simulink model "Loop_model"  (R2023b)
settings: Solver=ode5  StartTime=0.0  StopTime=1e4  RelTol=1e-3
values from neighbouring files (symbols this model uses):
  a = 6851.22197053    [IGRF13_2020.mat]    (also in complete_model.m; complete_model_main.m; loop_model.m; orbit_plot_report.m)
  alpha1 = 0.4    [IGRF13_2020.mat]    (also in complete_model.m = 0.05; complete_model_main.m; loop_model.m)
  alpha2 = 0.1    [IGRF13_2020.mat]    (also in complete_model.m = 0.15; complete_model_main.m; loop_model.m)
  alpha3 = 0.5    [IGRF13_2020.mat]    (also in complete_model.m = 0.8; complete_model_main.m; loop_model.m)
  bias_earth = [0.0282799758328 0.672423061801 0.739626573972]    [IGRF13_2020.mat]    (also in bias_good.mat = [0.12529783722 0.977879152241 0.167489747749]; complete_model.m = bias_earth./norm(bias_earth); loop_model.m = bias_earth./norm(bias_earth))
  bias_mag = [0.139359936806 0.414251479478 0.899430108326]    [IGRF13_2020.mat]    (also in bias_good.mat = [0.633137130131 0.601746707773 0.486865766031]; complete_model.m = bias_mag./norm(bias_mag); loop_model.m = bias_mag./norm(bias_mag))
  bias_sun = [0.56325131841 0.682189313334 0.466224938288]    [IGRF13_2020.mat]    (also in bias_good.mat = [0.711264013876 0.679091205187 0.181490048217]; complete_model.m = bias_sun./norm(bias_sun); loop_model.m = bias_sun./norm(bias_sun))
  e = 0.00183012221618    [IGRF13_2020.mat]    (also in complete_model.m; complete_model_main.m; loop_model.m; orbit_plot_report.m)
  FOV_earth = 0.575958653158    [IGRF13_2020.mat]    (also in complete_model.m = deg2rad(33); complete_model_main.m = deg2rad(33); loop_model.m = deg2rad(33))
  freq_acds = 30    [IGRF13_2020.mat]    (also in complete_model.m; loop_model.m)
  freq_act = 30    [IGRF13_2020.mat]    (also in complete_model.m; complete_model_main.m = 5; loop_model.m)
  freq_earth = 30    [IGRF13_2020.mat]    (also in complete_model.m; complete_model_main.m = 5; loop_model.m)
  freq_mag = 30    [IGRF13_2020.mat]    (also in complete_model.m; complete_model_main.m = 5; loop_model.m)
  freq_sun = 30    [IGRF13_2020.mat]    (also in complete_model.m; complete_model_main.m = 5; loop_model.m)
  gh = [-29404.8 -1450.9 4652.5 -2499.6 2982 -2991.6 1677 -734.6 1363.2 -2381.2 -82.1 1236.2 ... (195 elements, 195x1)]    [IGRF13_2020.mat]
  H0 = 2.98059244128e-05    [IGRF13_2020.mat]    (also in complete_model.m = sqrt(g01^2+g11^2+h11^2)*1e-9; complete_model_main.m = sqrt(g01^2+g11^2+h11^2)*1e-9; loop_model.m = sqrt(g01^2+g11^2+h11^2)*1e-9)
  I_ext = [22.9724026819  0  0; 0  7.77699984285  0; 0  0  23.1895034219]    [IGRF13_2020.mat]    (also in complete_model.m = diag([I1_ext I2_ext I3_ext]); loop_model.m = diag([I1_ext I2_ext I3_ext]))
  I_retr = [8.16666666667  0  0; 0  8.16666666667  0; 0  0  8.16666666667]    [IGRF13_2020.mat]    (also in complete_model.m = diag([I1_retr I2_retr I3_retr]); loop_model.m = diag([I1_retr I2_retr I3_retr]))
  I_wheel = 0.00636619772368    [IGRF13_2020.mat]    (also in complete_model.m; loop_model.m)
  Iinv_ext = [0.0435304923845  0  0; 0  0.128584289598  0; 0  0  0.0431229587718]    [IGRF13_2020.mat]    (also in complete_model.m = I_ext\eye(3); loop_model.m = I_ext\eye(3))
  Iinv_retr = [0.122448979592  0  0; 0  0.122448979592  0; 0  0  0.122448979592]    [IGRF13_2020.mat]    (also in complete_model.m = I_retr\eye(3); loop_model.m = I_retr\eye(3))
  incl = 0.200712863979    [IGRF13_2020.mat]    (also in complete_model.m = deg2rad(11.5); complete_model_main.m = deg2rad(11.5); loop_model.m = deg2rad(11.5))
  jb = [0.01 0.05 0.01]    [IGRF13_2020.mat]    (also in complete_model.m = [0.01; 0.05; 0.01]; complete_model_main.m = [0.01; 0.05; 0.01]; loop_model.m = [0.01; 0.05; 0.01])
  k_gain = 0.0363323388759    [IGRF13_2020.mat]    (also in complete_model.m = (4*pi/T) * (1 + sin(chsi)) * I1_retr; complete_model_main.m = (4*pi/T) * (1 + sin(chsi)) * min([I1, I2, I3]); loop_model.m = (4*pi/T) * (1 + sin(chsi)) * I1_retr)
  max_dip = 15    [IGRF13_2020.mat]    (also in complete_model.m; complete_model_main.m = 150; loop_model.m)
  max_hdot = 0.1    [IGRF13_2020.mat]    (also in complete_model.m; loop_model.m)
  mu = 398600.433    [IGRF13_2020.mat]    (also in complete_model.m = astroConstants(13); complete_model_main.m = astroConstants(13); loop_model.m = astroConstants(13); orbit_plot_report.m = astroConstants(13))
  n = 0.00111331183439    [IGRF13_2020.mat]    (also in complete_model.m = sqrt(mu/a^3); complete_model_main.m = sqrt(mu/a^3); loop_model.m = sqrt(mu/a^3); orbit_plot_report.m = sqrt(mu/a^3))
  noise_sd_mag = 1.18e-09    [IGRF13_2020.mat]    (also in complete_model.m; loop_model.m)
  omega0 = [0.06 0.06 0.06]    [IGRF13_2020.mat]    (also in complete_model.m = -0.06 + 0.12 * rand(3,1); complete_model_main.m = [0.01; 0.01; 0.01]*6; init_cond.mat = [-0.0472016675783 0.0554277697026 -0.0594438931039]; loop_model.m = 0.06 * ones(3,1))
  omegaE = 7.27220521664e-05    [IGRF13_2020.mat]    (also in complete_model.m = deg2rad(15)/3600; complete_model_main.m = deg2rad(15)/3600; loop_model.m = deg2rad(15)/3600)
  rs = [-16878165.0145 -134206589.72 -58177126.6728]    [IGRF13_2020.mat]    (also in complete_model.m = -rr; complete_model_main.m = -rr; loop_model.m = -rr; orbit_plot_report.m = -rr)
  Rt = 6371.01    [IGRF13_2020.mat]    (also in Terra_3D.m = 6378.1363; complete_model.m = astroConstants(23); complete_model_main.m = astroConstants(23); loop_model.m = astroConstants(23))
  s0 = [6.01405730572 3.04970514452 5.02831048374]    [IGRF13_2020.mat]    (also in buonnatale.mat = [2.59731710564 0.831637671153 -2.52872821404]; complete_model.m = 2*pi*rand(3,1); complete_model_main.m = -pi + 2 * pi * rand(3,1); init_cond.mat = [4.86890604626 5.13526758752 5.45816980916])
  tol = 0.2    [IGRF13_2020.mat]    (also in complete_model.m; complete_model_main.m; loop_model.m)
  w_sat = 628.318530718    [IGRF13_2020.mat]    (also in complete_model.m; loop_model.m)
undefined symbols (not defined in the file or in its folder): DiscIntNeverNeededParam, flag_h, magnitude, s_h, s_m, s_s, v_h, v_m, v_s
libraries: simulink x16, vrlib x9, matrix_library x7, cstextras x3, simulink_extras x1
(part 3 of 3)

== system Loop_model/Control/Slew Maneuver/Control Logic/Subsystem1 ==
  B_m : Inport
  u : Inport  Port=2
  Enable : EnablePort
  Assembly Matrix : Subsystem
  Constant : Constant  Value=0
  Constant1 : Constant  Value=0
  MATLAB Function : MATLAB Function  TreatAsAtomicUnit=on
  Selector : Selector  InputPortWidth=3  IndexOptions=Index vector (dialog)  Indices=2  OutputSizes=1
  Selector1 : Selector  InputPortWidth=3  IndexOptions=Index vector (dialog)  Indices=3  OutputSizes=1
  Selector2 : Selector  InputPortWidth=3  IndexOptions=Index vector (dialog)  Indices=1  OutputSizes=1
  Vector Concatenate : Concatenate  NumInputs=5
  Out1 : Outport
  wires:
  Assembly Matrix/1("Matrix ") -> MATLAB Function/1(A)
  B_m/1 -> Assembly Matrix/1(B_m)
  Selector1/1 -> Vector Concatenate/3
  Selector/1 -> Vector Concatenate/2
  Constant/1 -> Vector Concatenate/1
  Selector2/1 -> Vector Concatenate/4
  Constant1/1 -> Vector Concatenate/5
  MATLAB Function/1(x) -> Selector/1, Selector2/1, Selector1/1
  Vector Concatenate/1 -> Out1/1
  u/1 -> MATLAB Function/2(b)

== system Loop_model/Control/Slew Maneuver/compute alphadots/Discrete Derivative ==
  note: ( U(k) - U(k-1) )
  note: U(k)
  U : Inport
  Data Type Duplicate : DataTypeDuplicate  DisableCoverage=on  NumInputPorts=3
  Diff : Sum  Description=Add in CPU  Inputs=+-  OutMin=OutMin  OutMax=OutMax  OutDataTypeStr=diffDT
  TSamp : SampleTimeMath  DisableCoverage=on  TsampMathOp=/  weightValue=inverseGainval  TsampMathImp=Offline Scaling Adjustment
  UD : UnitDelay  Description=Store in Global RAM  DisableCoverage=on  InitialCondition=ICPrevScaledInput  SampleTime=-1  HasFrameUpgradeWarning=on
  Y : Outport  OutMin=OutMin  OutMax=OutMax  InitialOutput=0
  wires:
  U/1 -> TSamp/1
  UD/1 -> Diff/2, Data Type Duplicate/3  "U(k-1)"
  Diff/1 -> Y/1, Data Type Duplicate/1
  TSamp/1 -> UD/1, Diff/1, Data Type Duplicate/2

== system Loop_model/Control/Slew Maneuver/compute alphadots/Discrete Varying Lowpass ==
  u : Inport
  frequency : Inport  Port=2
  FOS : cstextras/DiscreteFirstOrderSection  VariantControl=(default)  Ts=Ts  w0=w0
  y : Outport  VectorParamsAs1DForOutWhenUnconnected=off
  wires:
  u/1 -> FOS/1
  frequency/1 -> FOS/2
  FOS/1 -> y/1

== system Loop_model/Control/Slew Maneuver/compute alphadots/Invert ==
  Matrix : Inport  PortDimensions=[3 3]
  Assertion : Assertion  AssertionFailFcn="disp('Matrix is singular.  No matrix inverse.')"
  Determinant of 3x3 Matrix : Subsystem
      settings: LibrarySourceBlock=|
      | sharedutil/Determinant of
      | 3x3 Matrix
  Product : Product  Inputs=/  Multiplication=Matrix(*)  SaturateOnIntegerOverflow=on  OutDataTypeStr=Inherit: Same as first input
  Matrix' : Outport  PortDimensions=[3 3]  VectorParamsAs1DForOutWhenUnconnected=off
  wires:
  Determinant of 3x3 Matrix/1(det) -> Assertion/1
  Product/1 -> Matrix'/1
  Matrix/1 -> Product/1, Determinant of 3x3 Matrix/1(Matrix)

== system Loop_model/Environment/Magnetic Field/compute Bn/compute m ==
  Clock : Clock
  Constant : Constant  Value=incl
  Constant1 : Constant  Value=omegaE
  Cos : Trigonometry  Operator=cos
  Cos1 : Trigonometry  Operator=cos
  Product : Product
  Product1 : Product
  Product2 : Product
  Scope : Scope
  Sin : Trigonometry
  Sin1 : Trigonometry
  Vector Concatenate : Concatenate  NumInputs=3
  m : Outport
  wires:
  Sin1/1 -> Product2/1
  Clock/1 -> Product/1
  Cos1/1 -> Product1/1
  Constant1/1 -> Product/2
  Product2/1 -> Vector Concatenate/2
  Sin/1 -> Product2/2, Product1/2
  Product/1 -> Sin1/1, Cos1/1
  Product1/1 -> Vector Concatenate/1
  Constant/1 -> Cos/1, Sin/1
  Vector Concatenate/1 -> m/1, Scope/1
  Cos/1 -> Vector Concatenate/3

== system Loop_model/Environment/Magnetic Field/compute Bn/norm ==
  rN : Inport
  Dot Product : DotProduct  OutDataTypeStr=Inherit: Inherit via internal rule
  Sqrt : Sqrt
  Out1 : Outport
  wires:
  rN/1 -> Dot Product/1, Dot Product/2
  Dot Product/1 -> Sqrt/1
  Sqrt/1 -> Out1/1

== system Loop_model/Kinematics/Kinematics 312/Euler angles/Subsystem ==
  In1 : Inport
  In2 : Inport  Port=2
  In3 : Inport  Port=3
  Cos : Trigonometry  Operator=cos
  Product : Product
  Product1 : Product
  Sin : Trigonometry
  Sum : Sum
  Out1 : Outport
  wires:
  In3/1 -> Sin/1, Cos/1
  In1/1 -> Product/1
  Cos/1 -> Product/2
  Sin/1 -> Product1/1
  In2/1 -> Product1/2
  Product/1 -> Sum/1
  Product1/1 -> Sum/2
  Sum/1 -> Out1/1

== system Loop_model/Kinematics/Kinematics 312/Euler angles/Subsystem1 ==
  In1 : Inport
  In2 : Inport  Port=2
  In3 : Inport  Port=3
  Cos : Trigonometry  Operator=cos
  Product : Product
  Product1 : Product
  Sin : Trigonometry
  Sum : Sum
  Out1 : Outport
  wires:
  Sum/1 -> Out1/1
  Product1/1 -> Sum/2
  Product/1 -> Sum/1
  In2/1 -> Product1/2
  Sin/1 -> Product1/1
  Cos/1 -> Product/2
  In1/1 -> Product/1
  In3/1 -> Cos/1, Sin/1

== system Loop_model/Kinematics/Kinematics 312/Euler angles/Subsystem2 ==
  In1 : Inport
  In2 : Inport  Port=2
  In3 : Inport  Port=3
  Cos : Trigonometry  Operator=cos
  Product : Product
  Product1 : Product
  Sin : Trigonometry
  Sum : Sum
  Out1 : Outport
  wires:
  In3/1 -> Sin/1, Cos/1
  In1/1 -> Product/1
  Cos/1 -> Product/2
  Sin/1 -> Product1/1
  In2/1 -> Product1/2
  Product/1 -> Sum/1
  Product1/1 -> Sum/2
  Sum/1 -> Out1/1

== system Loop_model/Kinematics/Kinematics 312/s_312 - A/R1 ==
  x : Inport
  Constant : Constant  Value=[1; 0; 0]
  Constant1 : Constant  Value=0
  Cos : Trigonometry  Operator=cos
  Gain : Gain  Gain=-1
  Matrix Concatenate : Concatenate  NumInputs=3  Mode=Multidimensional array  ConcatenateDimension=2
  Sin : Trigonometry
  Vector Concatenate : Concatenate  NumInputs=3
  Vector Concatenate1 : Concatenate  NumInputs=3
  R1 : Outport
  wires:
  Matrix Concatenate/1 -> R1/1
  x/1 -> Cos/1, Sin/1
  Vector Concatenate1/1 -> Matrix Concatenate/2
  Constant/1 -> Matrix Concatenate/1
  Vector Concatenate/1 -> Matrix Concatenate/3
  Constant1/1 -> Vector Concatenate/1, Vector Concatenate1/1
  Cos/1 -> Vector Concatenate/3, Vector Concatenate1/2
  Gain/1 -> Vector Concatenate1/3
  Sin/1 -> Vector Concatenate/2, Gain/1

== system Loop_model/Kinematics/Kinematics 312/s_312 - A/R2 ==
  x : Inport
  Constant : Constant  Value=[0; 1; 0]
  Constant1 : Constant  Value=0
  Cos : Trigonometry  Operator=cos
  Gain : Gain  Gain=-1
  Matrix Concatenate : Concatenate  NumInputs=3  Mode=Multidimensional array  ConcatenateDimension=2
  Sin : Trigonometry
  Vector Concatenate : Concatenate  NumInputs=3
  Vector Concatenate1 : Concatenate  NumInputs=3
  R2 : Outport
  wires:
  Vector Concatenate/1 -> Matrix Concatenate/1
  x/1 -> Sin/1, Cos/1
  Matrix Concatenate/1 -> R2/1
  Constant/1 -> Matrix Concatenate/2
  Vector Concatenate1/1 -> Matrix Concatenate/3
  Constant1/1 -> Vector Concatenate/2, Vector Concatenate1/2
  Cos/1 -> Vector Concatenate1/3, Vector Concatenate/1
  Sin/1 -> Gain/1, Vector Concatenate/3
  Gain/1 -> Vector Concatenate1/1

== system Loop_model/Kinematics/Kinematics 312/s_312 - A/R3 ==
  x : Inport
  Constant : Constant  Value=[0; 0; 1]
  Constant1 : Constant  Value=0
  Cos : Trigonometry  Operator=cos
  Gain : Gain  Gain=-1
  Matrix Concatenate : Concatenate  NumInputs=3  Mode=Multidimensional array  ConcatenateDimension=2
  Sin : Trigonometry
  Vector Concatenate : Concatenate  NumInputs=3
  Vector Concatenate1 : Concatenate  NumInputs=3
  R3 : Outport
  wires:
  Vector Concatenate/1 -> Matrix Concatenate/1
  Sin/1 -> Vector Concatenate1/1, Gain/1
  Cos/1 -> Vector Concatenate1/2, Vector Concatenate/1
  Constant/1 -> Matrix Concatenate/3
  Gain/1 -> Vector Concatenate/2
  Vector Concatenate1/1 -> Matrix Concatenate/2
  x/1 -> Sin/1, Cos/1
  Constant1/1 -> Vector Concatenate/3, Vector Concatenate1/3
  Matrix Concatenate/1 -> R3/1

== system Loop_model/Kinematics/Kinematics 312/s_313 - A/R1 ==
  x : Inport
  Constant : Constant  Value=[1; 0; 0]
  Constant1 : Constant  Value=0
  Cos : Trigonometry  Operator=cos
  Gain : Gain  Gain=-1
  Matrix Concatenate : Concatenate  NumInputs=3  Mode=Multidimensional array  ConcatenateDimension=2
  Sin : Trigonometry
  Vector Concatenate : Concatenate  NumInputs=3
  Vector Concatenate1 : Concatenate  NumInputs=3
  R1 : Outport
  wires:
  Sin/1 -> Gain/1, Vector Concatenate/2
  Gain/1 -> Vector Concatenate1/3
  Cos/1 -> Vector Concatenate1/2, Vector Concatenate/3
  Constant1/1 -> Vector Concatenate1/1, Vector Concatenate/1
  Vector Concatenate/1 -> Matrix Concatenate/3
  Constant/1 -> Matrix Concatenate/1
  Vector Concatenate1/1 -> Matrix Concatenate/2
  x/1 -> Sin/1, Cos/1
  Matrix Concatenate/1 -> R1/1

== system Loop_model/Kinematics/Kinematics 312/s_313 - A/R3_1 ==
  x : Inport
  Constant : Constant  Value=[0; 0; 1]
  Constant1 : Constant  Value=0
  Cos : Trigonometry  Operator=cos
  Gain : Gain  Gain=-1
  Matrix Concatenate : Concatenate  NumInputs=3  Mode=Multidimensional array  ConcatenateDimension=2
  Sin : Trigonometry
  Vector Concatenate : Concatenate  NumInputs=3
  Vector Concatenate1 : Concatenate  NumInputs=3
  R3 : Outport
  wires:
  Matrix Concatenate/1 -> R3/1
  Constant1/1 -> Vector Concatenate1/3, Vector Concatenate/3
  x/1 -> Cos/1, Sin/1
  Vector Concatenate1/1 -> Matrix Concatenate/2
  Gain/1 -> Vector Concatenate/2
  Constant/1 -> Matrix Concatenate/3
  Cos/1 -> Vector Concatenate/1, Vector Concatenate1/2
  Sin/1 -> Gain/1, Vector Concatenate1/1
  Vector Concatenate/1 -> Matrix Concatenate/1

== system Loop_model/Kinematics/Kinematics 312/s_313 - A/R3_2 ==
  x : Inport
  Constant : Constant  Value=[0; 0; 1]
  Constant1 : Constant  Value=0
  Cos : Trigonometry  Operator=cos
  Gain : Gain  Gain=-1
  Matrix Concatenate : Concatenate  NumInputs=3  Mode=Multidimensional array  ConcatenateDimension=2
  Sin : Trigonometry
  Vector Concatenate : Concatenate  NumInputs=3
  Vector Concatenate1 : Concatenate  NumInputs=3
  R3 : Outport
  wires:
  Vector Concatenate/1 -> Matrix Concatenate/1
  Sin/1 -> Vector Concatenate1/1, Gain/1
  Cos/1 -> Vector Concatenate1/2, Vector Concatenate/1
  Constant/1 -> Matrix Concatenate/3
  Gain/1 -> Vector Concatenate/2
  Vector Concatenate1/1 -> Matrix Concatenate/2
  x/1 -> Sin/1, Cos/1
  Constant1/1 -> Vector Concatenate/3, Vector Concatenate1/3
  Matrix Concatenate/1 -> R3/1

== system Loop_model/Kinematics/Kinematics 313/Euler angles/Subsystem ==
  In1 : Inport
  In2 : Inport  Port=2
  In3 : Inport  Port=3
  Cos : Trigonometry  Operator=cos
  Product : Product
  Product1 : Product
  Sin : Trigonometry
  Sum : Sum
  Out1 : Outport
  wires:
  Sum/1 -> Out1/1
  Product1/1 -> Sum/2
  Product/1 -> Sum/1
  In2/1 -> Product1/2
  Sin/1 -> Product1/1
  Cos/1 -> Product/2
  In1/1 -> Product/1
  In3/1 -> Cos/1, Sin/1

== system Loop_model/Kinematics/Kinematics 313/Euler angles/Subsystem1 ==
  In1 : Inport
  In2 : Inport  Port=2
  In3 : Inport  Port=3
  Cos : Trigonometry  Operator=cos
  Product : Product
  Product1 : Product
  Sin : Trigonometry
  Sum : Sum
  Out1 : Outport
  wires:
  In3/1 -> Sin/1, Cos/1
  In1/1 -> Product/1
  Cos/1 -> Product/2
  Sin/1 -> Product1/1
  In2/1 -> Product1/2
  Product/1 -> Sum/1
  Product1/1 -> Sum/2
  Sum/1 -> Out1/1

== system Loop_model/Kinematics/Kinematics 313/Euler angles/Subsystem2 ==
  In1 : Inport
  In2 : Inport  Port=2
  In3 : Inport  Port=3
  Cos : Trigonometry  Operator=cos
  Product : Product
  Product1 : Product
  Sin : Trigonometry
  Sum : Sum
  Out1 : Outport
  wires:
  Sum/1 -> Out1/1
  Product1/1 -> Sum/2
  Product/1 -> Sum/1
  In2/1 -> Product1/2
  Sin/1 -> Product1/1
  Cos/1 -> Product/2
  In1/1 -> Product/1
  In3/1 -> Cos/1, Sin/1

== system Loop_model/Kinematics/Kinematics 313/s_312 - A/R1 ==
  x : Inport
  Constant : Constant  Value=[1; 0; 0]
  Constant1 : Constant  Value=0
  Cos : Trigonometry  Operator=cos
  Gain : Gain  Gain=-1
  Matrix Concatenate : Concatenate  NumInputs=3  Mode=Multidimensional array  ConcatenateDimension=2
  Sin : Trigonometry
  Vector Concatenate : Concatenate  NumInputs=3
  Vector Concatenate1 : Concatenate  NumInputs=3
  R1 : Outport
  wires:
  Matrix Concatenate/1 -> R1/1
  x/1 -> Cos/1, Sin/1
  Vector Concatenate1/1 -> Matrix Concatenate/2
  Constant/1 -> Matrix Concatenate/1
  Vector Concatenate/1 -> Matrix Concatenate/3
  Constant1/1 -> Vector Concatenate/1, Vector Concatenate1/1
  Cos/1 -> Vector Concatenate/3, Vector Concatenate1/2
  Gain/1 -> Vector Concatenate1/3
  Sin/1 -> Vector Concatenate/2, Gain/1

== system Loop_model/Kinematics/Kinematics 313/s_312 - A/R2 ==
  x : Inport
  Constant : Constant  Value=[0; 1; 0]
  Constant1 : Constant  Value=0
  Cos : Trigonometry  Operator=cos
  Gain : Gain  Gain=-1
  Matrix Concatenate : Concatenate  NumInputs=3  Mode=Multidimensional array  ConcatenateDimension=2
  Sin : Trigonometry
  Vector Concatenate : Concatenate  NumInputs=3
  Vector Concatenate1 : Concatenate  NumInputs=3
  R2 : Outport
  wires:
  Vector Concatenate/1 -> Matrix Concatenate/1
  x/1 -> Sin/1, Cos/1
  Matrix Concatenate/1 -> R2/1
  Constant/1 -> Matrix Concatenate/2
  Vector Concatenate1/1 -> Matrix Concatenate/3
  Constant1/1 -> Vector Concatenate/2, Vector Concatenate1/2
  Cos/1 -> Vector Concatenate1/3, Vector Concatenate/1
  Sin/1 -> Gain/1, Vector Concatenate/3
  Gain/1 -> Vector Concatenate1/1

== system Loop_model/Kinematics/Kinematics 313/s_312 - A/R3 ==
  x : Inport
  Constant : Constant  Value=[0; 0; 1]
  Constant1 : Constant  Value=0
  Cos : Trigonometry  Operator=cos
  Gain : Gain  Gain=-1
  Matrix Concatenate : Concatenate  NumInputs=3  Mode=Multidimensional array  ConcatenateDimension=2
  Sin : Trigonometry
  Vector Concatenate : Concatenate  NumInputs=3
  Vector Concatenate1 : Concatenate  NumInputs=3
  R3 : Outport
  wires:
  Vector Concatenate/1 -> Matrix Concatenate/1
  Sin/1 -> Vector Concatenate1/1, Gain/1
  Cos/1 -> Vector Concatenate1/2, Vector Concatenate/1
  Constant/1 -> Matrix Concatenate/3
  Gain/1 -> Vector Concatenate/2
  Vector Concatenate1/1 -> Matrix Concatenate/2
  x/1 -> Sin/1, Cos/1
  Constant1/1 -> Vector Concatenate/3, Vector Concatenate1/3
  Matrix Concatenate/1 -> R3/1

== system Loop_model/Kinematics/Kinematics 313/s_313 - A/R1 ==
  x : Inport
  Constant : Constant  Value=[1; 0; 0]
  Constant1 : Constant  Value=0
  Cos : Trigonometry  Operator=cos
  Gain : Gain  Gain=-1
  Matrix Concatenate : Concatenate  NumInputs=3  Mode=Multidimensional array  ConcatenateDimension=2
  Sin : Trigonometry
  Vector Concatenate : Concatenate  NumInputs=3
  Vector Concatenate1 : Concatenate  NumInputs=3
  R1 : Outport
  wires:
  Sin/1 -> Gain/1, Vector Concatenate/2
  Gain/1 -> Vector Concatenate1/3
  Cos/1 -> Vector Concatenate1/2, Vector Concatenate/3
  Constant1/1 -> Vector Concatenate1/1, Vector Concatenate/1
  Vector Concatenate/1 -> Matrix Concatenate/3
  Constant/1 -> Matrix Concatenate/1
  Vector Concatenate1/1 -> Matrix Concatenate/2
  x/1 -> Sin/1, Cos/1
  Matrix Concatenate/1 -> R1/1

== system Loop_model/Kinematics/Kinematics 313/s_313 - A/R3_1 ==
  x : Inport
  Constant : Constant  Value=[0; 0; 1]
  Constant1 : Constant  Value=0
  Cos : Trigonometry  Operator=cos
  Gain : Gain  Gain=-1
  Matrix Concatenate : Concatenate  NumInputs=3  Mode=Multidimensional array  ConcatenateDimension=2
  Sin : Trigonometry
  Vector Concatenate : Concatenate  NumInputs=3
  Vector Concatenate1 : Concatenate  NumInputs=3
  R3 : Outport
  wires:
  Matrix Concatenate/1 -> R3/1
  Constant1/1 -> Vector Concatenate1/3, Vector Concatenate/3
  x/1 -> Cos/1, Sin/1
  Vector Concatenate1/1 -> Matrix Concatenate/2
  Gain/1 -> Vector Concatenate/2
  Constant/1 -> Matrix Concatenate/3
  Cos/1 -> Vector Concatenate/1, Vector Concatenate1/2
  Sin/1 -> Gain/1, Vector Concatenate1/1
  Vector Concatenate/1 -> Matrix Concatenate/1

== system Loop_model/Kinematics/Kinematics 313/s_313 - A/R3_2 ==
  x : Inport
  Constant : Constant  Value=[0; 0; 1]
  Constant1 : Constant  Value=0
  Cos : Trigonometry  Operator=cos
  Gain : Gain  Gain=-1
  Matrix Concatenate : Concatenate  NumInputs=3  Mode=Multidimensional array  ConcatenateDimension=2
  Sin : Trigonometry
  Vector Concatenate : Concatenate  NumInputs=3
  Vector Concatenate1 : Concatenate  NumInputs=3
  R3 : Outport
  wires:
  Vector Concatenate/1 -> Matrix Concatenate/1
  Sin/1 -> Vector Concatenate1/1, Gain/1
  Cos/1 -> Vector Concatenate1/2, Vector Concatenate/1
  Constant/1 -> Matrix Concatenate/3
  Gain/1 -> Vector Concatenate/2
  Vector Concatenate1/1 -> Matrix Concatenate/2
  x/1 -> Sin/1, Cos/1
  Constant1/1 -> Vector Concatenate/3, Vector Concatenate1/3
  Matrix Concatenate/1 -> R3/1

== system Loop_model/Control/Slew Maneuver/Control Logic/Subsystem/Assembly Matrix ==
  Bm : Inport
  Constant : Constant  Value=0
  Constant1 : Constant
  Constant2 : Constant  Value=0
  Demux : Demux  Outputs=3
  Gain : Gain  Gain=-1
  Gain1 : Gain  Gain=-1
  Gain2 : Gain  Gain=-1
  Matrix Concatenate : Concatenate  NumInputs=3  Mode=Multidimensional array  ConcatenateDimension=2
  Vector Concatenate : Concatenate  NumInputs=3
  Vector Concatenate1 : Concatenate  NumInputs=3
  Vector Concatenate2 : Concatenate  NumInputs=3
  Matrix : Outport
  wires:
  Constant/1 -> Vector Concatenate/1
  Bm/1 -> Demux/1
  Gain/1 -> Vector Concatenate/2
  Demux/3 -> Vector Concatenate1/1, Gain/1
  Demux/2 -> Gain2/1, Vector Concatenate/3
  Constant1/1 -> Vector Concatenate1/2
  Gain1/1 -> Vector Concatenate1/3
  Demux/1 -> Vector Concatenate2/2, Gain1/1
  Gain2/1 -> Vector Concatenate2/1
  Constant2/1 -> Vector Concatenate2/3
  Vector Concatenate1/1 -> Matrix Concatenate/2
  Vector Concatenate/1 -> Matrix Concatenate/1
  Vector Concatenate2/1 -> Matrix Concatenate/3
  Matrix Concatenate/1 -> Matrix/1

== system Loop_model/Control/Slew Maneuver/Control Logic/Subsystem1/Assembly Matrix ==
  B_m : Inport
  Constant : Constant  Value=0
  Constant1 : Constant
  Demux : Demux  Outputs=3
  Gain : Gain  Gain=-1
  Gain1 : Gain  Gain=-1
  Gain2 : Gain  Gain=-1
  Matrix Concatenate : Concatenate  NumInputs=3  Mode=Multidimensional array  ConcatenateDimension=2
  Vector Concatenate : Concatenate  NumInputs=3
  Vector Concatenate1 : Concatenate  NumInputs=3
  Vector Concatenate2 : Concatenate  NumInputs=3
  "Matrix " : Outport
  wires:
  B_m/1 -> Demux/1
  Constant1/1 -> Vector Concatenate/1
  Gain/1 -> Vector Concatenate/2
  Demux/3 -> Gain/1, Vector Concatenate1/1
  Demux/2 -> Gain2/1, Vector Concatenate/3
  Gain1/1 -> Vector Concatenate1/3
  Demux/1 -> Gain1/1, Vector Concatenate2/2
  Constant/1 -> Vector Concatenate1/2, Vector Concatenate2/3
  Gain2/1 -> Vector Concatenate2/1
  Vector Concatenate1/1 -> Matrix Concatenate/2
  Vector Concatenate/1 -> Matrix Concatenate/1
  Vector Concatenate2/1 -> Matrix Concatenate/3
  Matrix Concatenate/1 -> "Matrix "/1

== system Loop_model/Control/Slew Maneuver/compute alphadots/Invert/Determinant of 3x3 Matrix ==
  Matrix : Inport  PortDimensions=[3 3]
  Product{,1..5} (6 alike) : Product  Inputs=1  SaturateOnIntegerOverflow=on  OutDataTypeStr=Inherit: Same as first input
  Reshape : Reshape  OutputDimensionality=Column vector (2-D)
  Sum : Sum  Inputs=+--++-  SaturateOnIntegerOverflow=on
  a(1,1),a(2,2),a(3,3) : Selector  InputPortWidth=9  IndexOptions=Index vector (dialog)  Indices=[1 5 9]  OutputSizes=1
  a(1,1),a(2,3),a(3,2) : Selector  InputPortWidth=9  IndexOptions=Index vector (dialog)  Indices=[1 6 8]  OutputSizes=1
  a(1,2),a(2,1),a(3,3) : Selector  InputPortWidth=9  IndexOptions=Index vector (dialog)  Indices=[2 4 9]  OutputSizes=1
  a(1,2),a(2,3),a(3,1) : Selector  InputPortWidth=9  IndexOptions=Index vector (dialog)  Indices=[3 4 8]  OutputSizes=1
  a(1,3),a(2,1),a(3,2) : Selector  InputPortWidth=9  IndexOptions=Index vector (dialog)  Indices=[2 6 7]  OutputSizes=1
  a(1,3),a(2,2),a(3,1) : Selector  InputPortWidth=9  IndexOptions=Index vector (dialog)  Indices=[3 5 7]  OutputSizes=1
  det : Outport  PortDimensions=1  VectorParamsAs1DForOutWhenUnconnected=off
  wires:
  Reshape/1 -> a(1,1),a(2,3),a(3,2)/1, a(1,1),a(2,2),a(3,3)/1, a(1,3),a(2,2),a(3,1)/1, a(1,3),a(2,1),a(3,2)/1, a(1,2),a(2,3),a(3,1)/1, a(1,2),a(2,1),a(3,3)/1
  Sum/1 -> det/1  "det(Matrix)"
  Matrix/1 -> Reshape/1
  Product5/1 -> Sum/6
  Product4/1 -> Sum/5
  Product3/1 -> Sum/4
  Product2/1 -> Sum/3
  Product1/1 -> Sum/2
  Product/1 -> Sum/1
  a(1,3),a(2,2),a(3,1)/1 -> Product5/1
  a(1,3),a(2,1),a(3,2)/1 -> Product4/1
  a(1,2),a(2,3),a(3,1)/1 -> Product3/1
  a(1,2),a(2,1),a(3,3)/1 -> Product2/1
  a(1,1),a(2,3),a(3,2)/1 -> Product1/1
  a(1,1),a(2,2),a(3,3)/1 -> Product/1

== matlab function Loop_model/Environment/Magnetic Field/MATLAB Function ==
  data: r input; B output; theta input; phi input; gh input
function B = calculateField(r, theta, phi, gh)

N = 13;         % Order of the field
lat = pi/2 - theta;
lon = phi;

R = 6371.2;     % Radius of Earth in IGRF
ratio = R / r;

sin_lat = sin(lat);
cos_lat = cos(lat);
sin_lon = sin(lon);
cos_lon = cos(lon);

npq = (N * (N+3)) / 2;

p = zeros(npq, 1);
p(1) = 2*sin_lat;
p(2) = 2*cos_lat;
p(3) = 4.5*sin_lat^2 - 1.5;
p(4) = 3*sqrt(3) * cos_lat * sin_lat;

q = zeros(npq, 1);
q(1) = -cos_lat;
q(2) = sin_lat;
q(3) = -3 * cos_lat * sin_lat;
q(4) = sqrt(3) * (sin_lat^2 - cos_lat^2);

sl = zeros(N+1, 1);
sl(1) = sin_lon;

cl = zeros(N+1, 1);
cl(1) = cos_lon;

Bx = 0; By = 0; Bz = 0;
l = 1; n = 0; m = 1;
fn = nan; rr = nan;

for k = 1:npq

    if n < m
        m = 0;
        n = n + 1;
        rr = ratio^(n+2);
        fn = n;
    end

    fm = m;

    if k >= 5

        if m == n
            a = sqrt(1 - 0.5/fm);
            j = k - n - 1;
            p(k) = (1 + 1/fm) * a * cos_lat * p(j);
            q(k) = a * (cos_lat * q(j) + sin_lat/fm * p(j));
            sl(m) = sl(m-1)*cl(1) + cl(m-1)*sl(1);
            cl(m) = cl(m-1)*cl(1) - sl(m-1)*sl(1);
        else
            a = sqrt(fn^2 - fm^2);
            b = sqrt((fn-1)^2 - fm^2) / a;
            c = (2*fn - 1) / a;
            ii = k - n;
            j = k - 2*n + 1;
            p(k) = (fn+1) * (c * sin_lat/fn * p(ii) - b/(fn-1) * p(j));
            q(k) = c * (sin_lat * q(ii) - cos_lat/fn * p(ii)) - b * q(j);
        end

    end

    a = rr * gh(l);
    
    if m == 0

        Bx = Bx + a*q(k);
        Bz = Bz - a*p(k);
        
        l = l + 1;

    else
        
        b = rr * gh(l+1);
        c = a*cl(m) + b*sl(m);
        Bx = Bx + c * q(k);
        Bz = Bz - c * p(k);
        
        if cos_lat > 0
            By = By + (a*sl(m) - b*cl(m)) * fm * p(k)/((fn+1) * cos_lat);
        else
            By = By + (a*sl(m) - b*cl(m)) * q(k) * sin_lat;
        end
        
        l = l + 2;

    end

    m = m + 1;

end

B_NED = [Bx; By; Bz] * 1e-9;

% Convert NED to ECEF
R = [-sin_lat * cos_lon,    -sin_lon,   -cos_lat * cos_lon;
     -sin_lat * sin_lon,    cos_lon,    -cos_lat * sin_lon;
     cos_lat,               0,          -sin_lat            ];

B = R * B_NED;

== matlab function Loop_model/Control/Slew Maneuver/Control Logic/Subsystem/MATLAB Function ==
  data: A input; x output; b input
function x = solve(A, b)

x = A \ b;

== matlab function Loop_model/Attitude Determination/Statistical Method/MATLAB Function ==
  data: A input; U output; V output
function [U,V] = SVD(A)

[U,~,V] = svd(A);

end

== matlab function Loop_model/Control/Slew Maneuver/Control Logic/Subsystem1/MATLAB Function ==
  data: A input; x output; b input
function x = solve(A, b)

x = A \ b;
